simulink model "punto3"  (R2020b)
settings: Solver=VariableStepAuto  StartTime=0.0  StopTime=0.045  RelTol=1e-3
values from neighbouring files (symbols this model uses):
  C = 4e-6    (= 4e-06)    [codigo.m]
  L = 10e-3    (= 0.01)    [codigo.m]
  R1 = 1e3    (= 1000)    [codigo.m]
  R2 = 2e3    (= 2000)    [codigo.m]
settings Model: Creator=Acer  LastModifiedBy=Acer

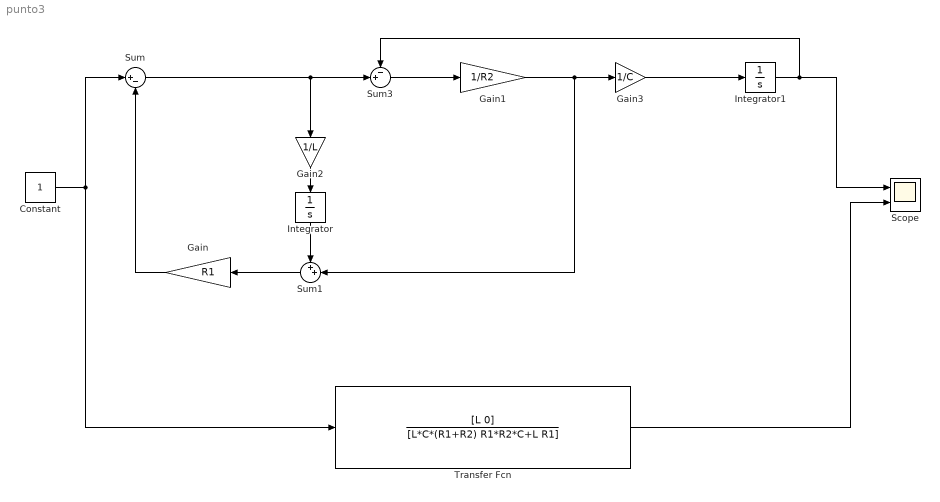
== system punto3 ==
  Constant : Constant
  Gain : Gain  Gain=R1
  Gain1 : Gain  Gain=1/R2
  Gain2 : Gain  Gain=1/L
  Gain3 : Gain  Gain=1/C
  Integrator : Integrator
  Integrator1 : Integrator
  Scope : Scope  NumInputPorts=2
  Sum : Sum  Inputs=|+-
  Sum1 : Sum  Inputs=++|
  Sum3 : Sum  Inputs=-+|
  Transfer Fcn : TransferFcn  Numerator=[L 0]  Denominator=[L*C*(R1+R2) R1*R2*C+L R1]
  wires:
  Constant/1 -> Transfer Fcn/1, Sum/1
  Sum/1 -> Gain2/1, Sum3/2
  Sum3/1 -> Gain1/1
  Gain1/1 -> Sum1/2, Gain3/1
  Gain3/1 -> Integrator1/1
  Integrator1/1 -> Scope/1, Sum3/1
  Transfer Fcn/1 -> Scope/2
  Gain/1 -> Sum/2
  Sum1/1 -> Gain/1
  Gain2/1 -> Integrator/1
  Integrator/1 -> Sum1/1
